simulink model "HAC_simulink"  (R2022b)
settings: Solver=VariableStepAuto  StartTime=0.0  StopTime=10.0  RelTol=1e-3
settings Model: Creator=doann  LastModifiedBy=doann

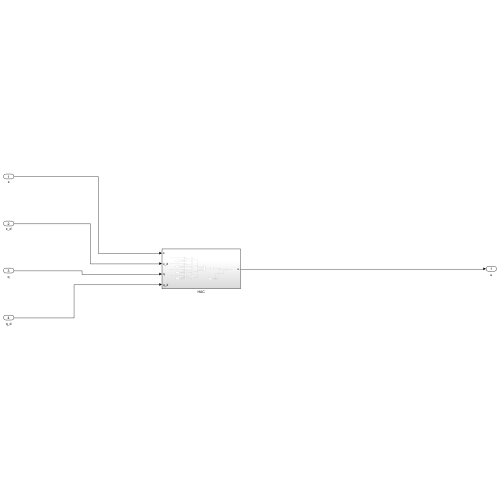
[thumbnail: Simulink's stored preview of the top-level diagram]
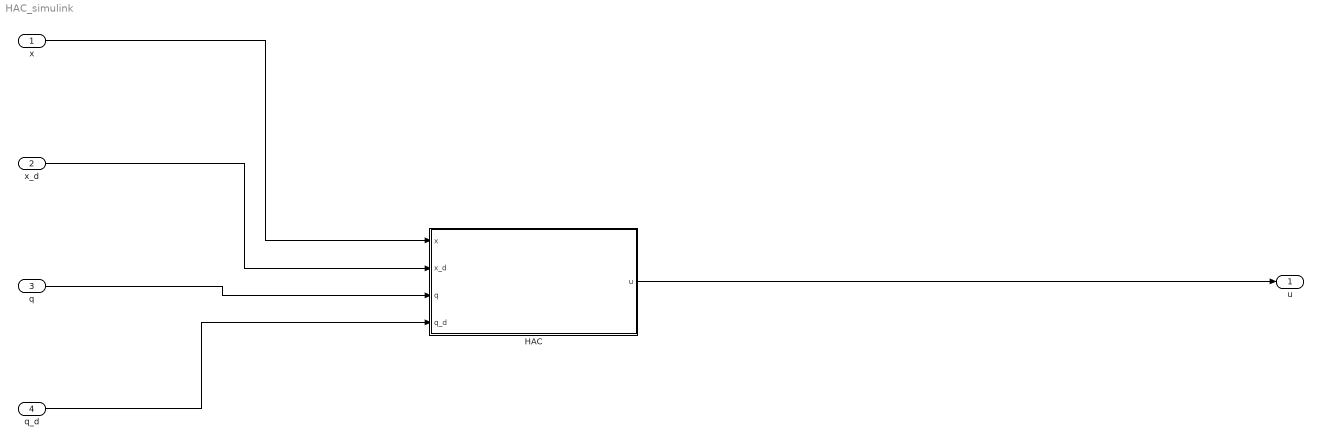
== system HAC_simulink ==
  x : Inport
  x_d : Inport  Port=2
  q : Inport  Port=3
  q_d : Inport  Port=4
  HAC : Subsystem
  u : Outport
  wires:
  x/1 -> HAC/1(x)
  x_d/1 -> HAC/2(x_d)
  q/1 -> HAC/3(q)
  q_d/1 -> HAC/4(q_d)
  HAC/1(u) -> u/1

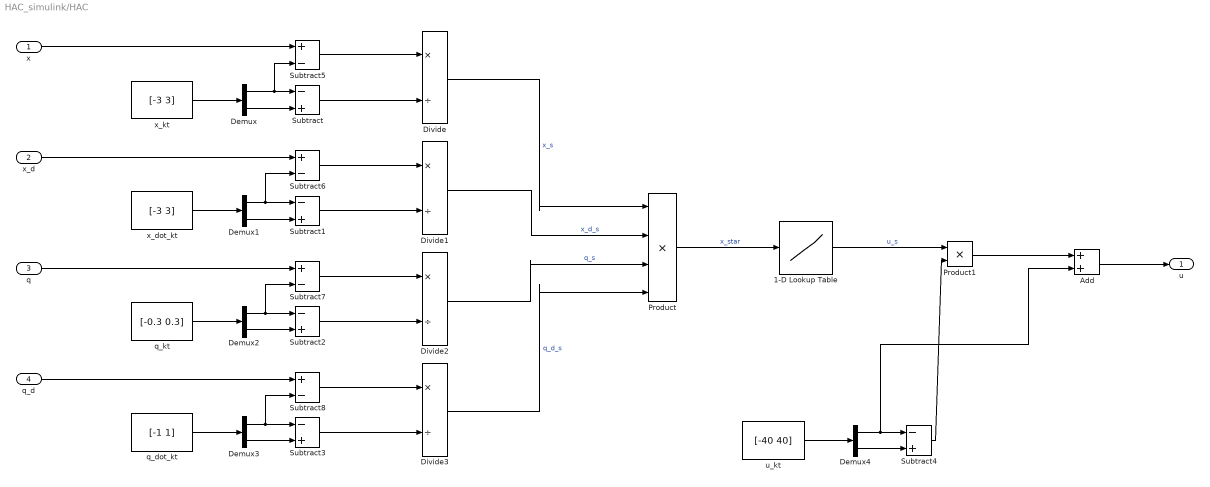
== system HAC_simulink/HAC ==
  x : Inport
  x_d : Inport  Port=2
  q : Inport  Port=3
  q_d : Inport  Port=4
  1-D Lookup Table : Lookup_n-D  NumberOfTableDimensions=1  BreakpointsForDimension1="[0 0.00390625 0.0078125\t0.01171875 0.015625\t0.0234375 0.03125\t0.03515625\t0.046875\t0.0625\t0.0703125\t0.09375\t0.10546875\t0.140625\t0.2109375\t0.31640625]"  Table="[0 0.15\t0.15\t0.25\t0.25\t0.375\t0.375\t0.5\t0.5\t0.5\t0.625\t0.625\t0.75\t0.75\t0.825\t0.825]"  InterpMethod=Akima spline  InternalRulePriority=Speed  RndMeth=Simplest
  Add : Sum
  Demux{,1..4} (5 alike) : Demux  Outputs=2
  Divide{,1..3} (4 alike) : Product  Inputs=*/
  Product : Product  Inputs=4
  Product1 : Product
  Subtract{,1..4} (5 alike) : Sum  Inputs=-+
  Subtract{5..8} (4 alike) : Sum  Inputs=+-
  q_dot_kt : Constant  Value=[-1 1]  VectorParams1D=off
  q_kt : Constant  Value=[-0.3 0.3]  VectorParams1D=off
  u_kt : Constant  Value=[-40 40]  VectorParams1D=off
  x_dot_kt : Constant  Value=[-3 3]  VectorParams1D=off
  x_kt : Constant  Value=[-3 3]  VectorParams1D=off
  u : Outport
  wires:
  Product1/1 -> Add/1
  Demux2/1 -> Subtract7/2, Subtract2/1
  Subtract7/1 -> Divide2/1
  Product/1 -> 1-D Lookup Table/1  "x_star"
  Demux3/2 -> Subtract3/2
  x_dot_kt/1 -> Demux1/1
  Subtract8/1 -> Divide3/1
  Divide1/1 -> Product/2  "x_d_s"
  Subtract6/1 -> Divide1/1
  1-D Lookup Table/1 -> Product1/1  "u_s"
  Demux1/1 -> Subtract6/2, Subtract1/1
  Divide2/1 -> Product/3  "q_s"
  Demux3/1 -> Subtract8/2, Subtract3/1
  x_d/1 -> Subtract6/1
  x_kt/1 -> Demux/1
  Subtract/1 -> Divide/2
  Subtract5/1 -> Divide/1
  Demux/1 -> Subtract5/2, Subtract/1
  Subtract3/1 -> Divide3/2
  Demux1/2 -> Subtract1/2
  Demux/2 -> Subtract/2
  u_kt/1 -> Demux4/1
  Subtract1/1 -> Divide1/2
  x/1 -> Subtract5/1
  Divide/1 -> Product/1  "x_s"
  q/1 -> Subtract7/1
  Add/1 -> u/1
  Divide3/1 -> Product/4  "q_d_s"
  q_d/1 -> Subtract8/1
  Demux4/1 -> Subtract4/1, Add/2
  Demux4/2 -> Subtract4/2
  Demux2/2 -> Subtract2/2
  q_dot_kt/1 -> Demux3/1
  q_kt/1 -> Demux2/1
  Subtract4/1 -> Product1/2
  Subtract2/1 -> Divide2/2
